simulink model "torqueBalancingYogaParametrizedForces2017"  (Simulink 9.0)
settings: Solver=FixedStepDiscrete  StartTime=0.0  StopTime="Config.SIMULATION_TIME "  FixedStep=Config.Ts  RelTol=1e-3  EnableMultiTasking=on
InitFcn:
  | cd(fileparts(which(bdroot)));
  | initTorqueBalancingYogaParametrized;
StopFcn:
  | cd(fileparts(which(bdroot)));
  | stopTorqueBalancingYoga;
undefined symbols (not defined in the file or in its folder): Config, delta_c, delta_x, delta_y, delta_z, DiscIntNeverNeededParam, Gain, Reg, ROBOT_DOF, ROBOT_DOF_FOR_SIMULINK, Sat, Sm
libraries: WBToolboxLibrary x85, simulink x4
(part 2 of 2)

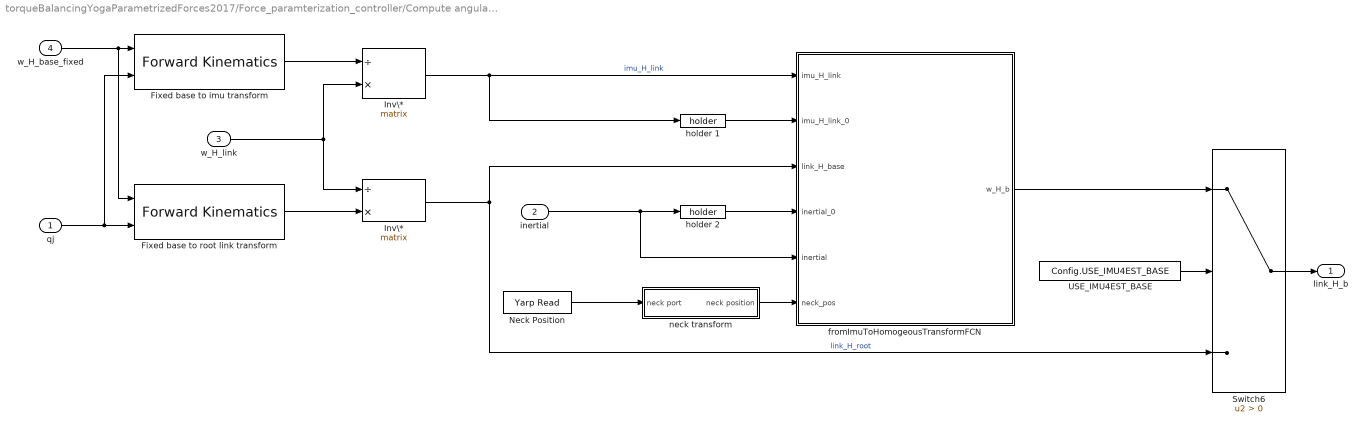
== system torqueBalancingYogaParametrizedForces2017/Force_paramterization_controller/Compute angular momentum integral/Compute base to fixed link transform/LFoot to base link transform  ==
  qj : Inport
  inertial : Inport  Port=2
  w_H_link : Inport  Port=3
  w_H_base_fixed : Inport  Port=4
  Fixed base to imu transform : WBToolboxLibrary/wholeBodyModel/Kinematics/Forward Kinematics  frameName=Frames.IMU
      settings: SourceProductName=Whole Body Toolbox
  Fixed base to root link transform : WBToolboxLibrary/wholeBodyModel/Kinematics/Forward Kinematics  frameName=Frames.BASE
      settings: SourceProductName=Whole Body Toolbox
  Inv\* : Product  Inputs=/*  Multiplication=Matrix(*)
  "Inv\\*  " : Product  Inputs=/*  Multiplication=Matrix(*)
  Neck Position : WBToolboxLibrary/Utilities/Yarp Read  portName=Ports.NECK_POS  signalSize=6  timeout=0.5  blocking=off  timestamp=off  autoconnect=on  errorOnConnection=off
      settings: SourceProductName=Whole Body Toolbox
  Switch6 : Switch  Criteria=u2 > Threshold
  USE_IMU4EST_BASE : Constant  Value=Config.USE_IMU4EST_BASE
  fromImuToHomogeousTransformFCN : MATLAB Function  TreatAsAtomicUnit=on
  holder 1 : WBToolboxLibrary/Utilities/holder 
      settings: SourceProductName=Whole Body Toolbox
  holder 2 : WBToolboxLibrary/Utilities/holder 
      settings: SourceProductName=Whole Body Toolbox
  neck transform : Subsystem
  link_H_b : Outport
  wires:
  Switch6/1 -> link_H_b/1
  "Inv\\*  "/1 -> Switch6/3, fromImuToHomogeousTransformFCN/3(link_H_base)  "link_H_root"
  USE_IMU4EST_BASE/1 -> Switch6/2
  Inv\*/1 -> fromImuToHomogeousTransformFCN/1(imu_H_link), holder 1/1  "imu_H_link"
  holder 2/1 -> fromImuToHomogeousTransformFCN/4(inertial_0)
  Fixed base to imu transform/1 -> Inv\*/1
  holder 1/1 -> fromImuToHomogeousTransformFCN/2(imu_H_link_0)
  qj/1 -> Fixed base to imu transform/2, Fixed base to root link transform/2
  fromImuToHomogeousTransformFCN/1(w_H_b) -> Switch6/1
  Fixed base to root link transform/1 -> "Inv\\*  "/2
  inertial/1 -> holder 2/1, fromImuToHomogeousTransformFCN/5(inertial)
  Neck Position/1 -> neck transform/1(neck port)
  neck transform/1(neck position) -> fromImuToHomogeousTransformFCN/6(neck_pos)
  w_H_link/1 -> "Inv\\*  "/1, Inv\*/2
  w_H_base_fixed/1 -> Fixed base to root link transform/1, Fixed base to imu transform/1

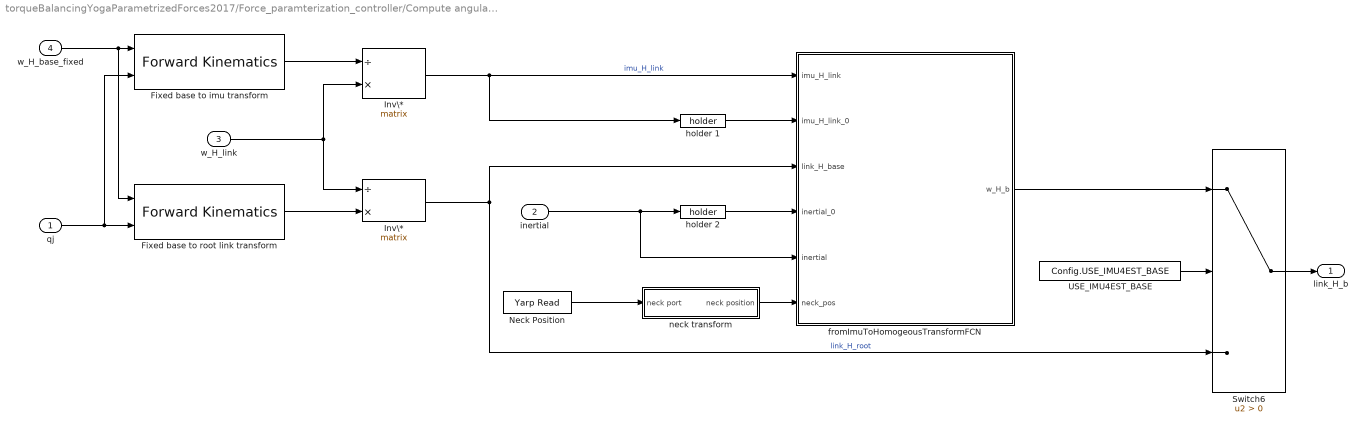
== system torqueBalancingYogaParametrizedForces2017/Force_paramterization_controller/Compute angular momentum integral/Compute base to fixed link transform/RFoot to base link transform ==
  qj : Inport
  inertial : Inport  Port=2
  w_H_link : Inport  Port=3
  w_H_base_fixed : Inport  Port=4
  Fixed base to imu transform : WBToolboxLibrary/wholeBodyModel/Kinematics/Forward Kinematics  frameName=Frames.IMU
      settings: SourceProductName=Whole Body Toolbox
  Fixed base to root link transform : WBToolboxLibrary/wholeBodyModel/Kinematics/Forward Kinematics  frameName=Frames.BASE
      settings: SourceProductName=Whole Body Toolbox
  Inv\* : Product  Inputs=/*  Multiplication=Matrix(*)
  "Inv\\*  " : Product  Inputs=/*  Multiplication=Matrix(*)
  Neck Position : WBToolboxLibrary/Utilities/Yarp Read  portName=Ports.NECK_POS  signalSize=6  timeout=0.5  blocking=off  timestamp=off  autoconnect=on  errorOnConnection=off
      settings: SourceProductName=Whole Body Toolbox
  Switch6 : Switch  Criteria=u2 > Threshold
  USE_IMU4EST_BASE : Constant  Value=Config.USE_IMU4EST_BASE
  fromImuToHomogeousTransformFCN : MATLAB Function  TreatAsAtomicUnit=on
  holder 1 : WBToolboxLibrary/Utilities/holder 
      settings: SourceProductName=Whole Body Toolbox
  holder 2 : WBToolboxLibrary/Utilities/holder 
      settings: SourceProductName=Whole Body Toolbox
  neck transform : Subsystem
  link_H_b : Outport
  wires:
  Switch6/1 -> link_H_b/1
  "Inv\\*  "/1 -> Switch6/3, fromImuToHomogeousTransformFCN/3(link_H_base)  "link_H_root"
  USE_IMU4EST_BASE/1 -> Switch6/2
  Inv\*/1 -> fromImuToHomogeousTransformFCN/1(imu_H_link), holder 1/1  "imu_H_link"
  holder 2/1 -> fromImuToHomogeousTransformFCN/4(inertial_0)
  Fixed base to imu transform/1 -> Inv\*/1
  holder 1/1 -> fromImuToHomogeousTransformFCN/2(imu_H_link_0)
  qj/1 -> Fixed base to imu transform/2, Fixed base to root link transform/2
  fromImuToHomogeousTransformFCN/1(w_H_b) -> Switch6/1
  Fixed base to root link transform/1 -> "Inv\\*  "/2
  inertial/1 -> holder 2/1, fromImuToHomogeousTransformFCN/5(inertial)
  Neck Position/1 -> neck transform/1(neck port)
  neck transform/1(neck position) -> fromImuToHomogeousTransformFCN/6(neck_pos)
  w_H_link/1 -> "Inv\\*  "/1, Inv\*/2
  w_H_base_fixed/1 -> Fixed base to root link transform/1, Fixed base to imu transform/1

== system torqueBalancingYogaParametrizedForces2017/Robot State and References/Internal Coordinator/Base to fixed_link/LFoot to base link transform  ==
  qj : Inport
  inertial : Inport  Port=2
  w_H_link : Inport  Port=3
  w_H_base_fixed : Inport  Port=4
  Fixed base to imu transform : WBToolboxLibrary/wholeBodyModel/Kinematics/Forward Kinematics  frameName=Frames.IMU
      settings: SourceProductName=Whole Body Toolbox
  Fixed base to root link transform : WBToolboxLibrary/wholeBodyModel/Kinematics/Forward Kinematics  frameName=Frames.BASE
      settings: SourceProductName=Whole Body Toolbox
  Inv\* : Product  Inputs=/*  Multiplication=Matrix(*)
  "Inv\\*  " : Product  Inputs=/*  Multiplication=Matrix(*)
  Neck Position : WBToolboxLibrary/Utilities/Yarp Read  portName=Ports.NECK_POS  signalSize=6  timeout=0.5  blocking=off  timestamp=off  autoconnect=on  errorOnConnection=off
      settings: SourceProductName=Whole Body Toolbox
  Switch6 : Switch  Criteria=u2 > Threshold
  USE_IMU4EST_BASE : Constant  Value=Config.USE_IMU4EST_BASE
  fromImuToHomogeousTransformFCN : MATLAB Function  TreatAsAtomicUnit=on
  holder 1 : WBToolboxLibrary/Utilities/holder 
      settings: SourceProductName=Whole Body Toolbox
  holder 2 : WBToolboxLibrary/Utilities/holder 
      settings: SourceProductName=Whole Body Toolbox
  neck transform : Subsystem
  link_H_b : Outport
  wires:
  Switch6/1 -> link_H_b/1
  "Inv\\*  "/1 -> Switch6/3, fromImuToHomogeousTransformFCN/3(link_H_base)  "link_H_root"
  USE_IMU4EST_BASE/1 -> Switch6/2
  Inv\*/1 -> fromImuToHomogeousTransformFCN/1(imu_H_link), holder 1/1  "imu_H_link"
  holder 2/1 -> fromImuToHomogeousTransformFCN/4(inertial_0)
  Fixed base to imu transform/1 -> Inv\*/1
  holder 1/1 -> fromImuToHomogeousTransformFCN/2(imu_H_link_0)
  qj/1 -> Fixed base to imu transform/2, Fixed base to root link transform/2
  fromImuToHomogeousTransformFCN/1(w_H_b) -> Switch6/1
  Fixed base to root link transform/1 -> "Inv\\*  "/2
  inertial/1 -> holder 2/1, fromImuToHomogeousTransformFCN/5(inertial)
  Neck Position/1 -> neck transform/1(neck port)
  neck transform/1(neck position) -> fromImuToHomogeousTransformFCN/6(neck_pos)
  w_H_link/1 -> "Inv\\*  "/1, Inv\*/2
  w_H_base_fixed/1 -> Fixed base to root link transform/1, Fixed base to imu transform/1

== system torqueBalancingYogaParametrizedForces2017/Robot State and References/Internal Coordinator/Compute State Velocity/Feet Jacobians ==
  qj : Inport
  w_H_b : Inport  Port=2
  Jacobian LFoot : WBToolboxLibrary/wholeBodyModel/Jacobians/Jacobian  frameName=Frames.LEFT_FOOT
      settings: SourceProductName=Whole Body Toolbox
  Jacobian RFoot : WBToolboxLibrary/wholeBodyModel/Jacobians/Jacobian  frameName=Frames.RIGHT_FOOT
      settings: SourceProductName=Whole Body Toolbox
  J_LFoot : Outport
  J_RFoot : Outport  Port=2
  wires:
  Jacobian LFoot/1 -> J_LFoot/1
  Jacobian RFoot/1 -> J_RFoot/1
  w_H_b/1 -> Jacobian RFoot/1, Jacobian LFoot/1
  qj/1 -> Jacobian LFoot/2, Jacobian RFoot/2

== system torqueBalancingYogaParametrizedForces2017/Robot State and References/State Machine Yoga/Compute State Velocity/Feet Jacobians ==
  qj : Inport
  w_H_b : Inport  Port=2
  Jacobian LFoot : WBToolboxLibrary/wholeBodyModel/Jacobians/Jacobian  frameName=Frames.LEFT_FOOT
      settings: SourceProductName=Whole Body Toolbox
  Jacobian RFoot : WBToolboxLibrary/wholeBodyModel/Jacobians/Jacobian  frameName=Frames.RIGHT_FOOT
      settings: SourceProductName=Whole Body Toolbox
  J_LFoot : Outport
  J_RFoot : Outport  Port=2
  wires:
  Jacobian LFoot/1 -> J_LFoot/1
  Jacobian RFoot/1 -> J_RFoot/1
  w_H_b/1 -> Jacobian RFoot/1, Jacobian LFoot/1
  qj/1 -> Jacobian LFoot/2, Jacobian RFoot/2

== system torqueBalancingYogaParametrizedForces2017/Robot State and References/State Machine Yoga/Compute base to fixed link transform/LFoot to base link transform  ==
  qj : Inport
  inertial : Inport  Port=2
  w_H_link : Inport  Port=3
  w_H_base_fixed : Inport  Port=4
  Fixed base to imu transform : WBToolboxLibrary/wholeBodyModel/Kinematics/Forward Kinematics  frameName=Frames.IMU
      settings: SourceProductName=Whole Body Toolbox
  Fixed base to root link transform : WBToolboxLibrary/wholeBodyModel/Kinematics/Forward Kinematics  frameName=Frames.BASE
      settings: SourceProductName=Whole Body Toolbox
  Inv\* : Product  Inputs=/*  Multiplication=Matrix(*)
  "Inv\\*  " : Product  Inputs=/*  Multiplication=Matrix(*)
  Neck Position : WBToolboxLibrary/Utilities/Yarp Read  portName=Ports.NECK_POS  signalSize=6  timeout=0.5  blocking=off  timestamp=off  autoconnect=on  errorOnConnection=off
      settings: SourceProductName=Whole Body Toolbox
  Switch6 : Switch  Criteria=u2 > Threshold
  USE_IMU4EST_BASE : Constant  Value=Config.USE_IMU4EST_BASE
  fromImuToHomogeousTransformFCN : MATLAB Function  TreatAsAtomicUnit=on
  holder 1 : WBToolboxLibrary/Utilities/holder 
      settings: SourceProductName=Whole Body Toolbox
  holder 2 : WBToolboxLibrary/Utilities/holder 
      settings: SourceProductName=Whole Body Toolbox
  neck transform : Subsystem
  link_H_b : Outport
  wires:
  Switch6/1 -> link_H_b/1
  "Inv\\*  "/1 -> Switch6/3, fromImuToHomogeousTransformFCN/3(link_H_base)  "link_H_root"
  USE_IMU4EST_BASE/1 -> Switch6/2
  Inv\*/1 -> fromImuToHomogeousTransformFCN/1(imu_H_link), holder 1/1  "imu_H_link"
  holder 2/1 -> fromImuToHomogeousTransformFCN/4(inertial_0)
  Fixed base to imu transform/1 -> Inv\*/1
  holder 1/1 -> fromImuToHomogeousTransformFCN/2(imu_H_link_0)
  qj/1 -> Fixed base to imu transform/2, Fixed base to root link transform/2
  fromImuToHomogeousTransformFCN/1(w_H_b) -> Switch6/1
  Fixed base to root link transform/1 -> "Inv\\*  "/2
  inertial/1 -> holder 2/1, fromImuToHomogeousTransformFCN/5(inertial)
  Neck Position/1 -> neck transform/1(neck port)
  neck transform/1(neck position) -> fromImuToHomogeousTransformFCN/6(neck_pos)
  w_H_link/1 -> "Inv\\*  "/1, Inv\*/2
  w_H_base_fixed/1 -> Fixed base to root link transform/1, Fixed base to imu transform/1

== system torqueBalancingYogaParametrizedForces2017/Robot State and References/State Machine Yoga/Compute base to fixed link transform/RFoot to base link transform ==
  qj : Inport
  inertial : Inport  Port=2
  w_H_link : Inport  Port=3
  w_H_base_fixed : Inport  Port=4
  Fixed base to imu transform : WBToolboxLibrary/wholeBodyModel/Kinematics/Forward Kinematics  frameName=Frames.IMU
      settings: SourceProductName=Whole Body Toolbox
  Fixed base to root link transform : WBToolboxLibrary/wholeBodyModel/Kinematics/Forward Kinematics  frameName=Frames.BASE
      settings: SourceProductName=Whole Body Toolbox
  Inv\* : Product  Inputs=/*  Multiplication=Matrix(*)
  "Inv\\*  " : Product  Inputs=/*  Multiplication=Matrix(*)
  Neck Position : WBToolboxLibrary/Utilities/Yarp Read  portName=Ports.NECK_POS  signalSize=6  timeout=0.5  blocking=off  timestamp=off  autoconnect=on  errorOnConnection=off
      settings: SourceProductName=Whole Body Toolbox
  Switch6 : Switch  Criteria=u2 > Threshold
  USE_IMU4EST_BASE : Constant  Value=Config.USE_IMU4EST_BASE
  fromImuToHomogeousTransformFCN : MATLAB Function  TreatAsAtomicUnit=on
  holder 1 : WBToolboxLibrary/Utilities/holder 
      settings: SourceProductName=Whole Body Toolbox
  holder 2 : WBToolboxLibrary/Utilities/holder 
      settings: SourceProductName=Whole Body Toolbox
  neck transform : Subsystem
  link_H_b : Outport
  wires:
  Switch6/1 -> link_H_b/1
  "Inv\\*  "/1 -> Switch6/3, fromImuToHomogeousTransformFCN/3(link_H_base)  "link_H_root"
  USE_IMU4EST_BASE/1 -> Switch6/2
  Inv\*/1 -> fromImuToHomogeousTransformFCN/1(imu_H_link), holder 1/1  "imu_H_link"
  holder 2/1 -> fromImuToHomogeousTransformFCN/4(inertial_0)
  Fixed base to imu transform/1 -> Inv\*/1
  holder 1/1 -> fromImuToHomogeousTransformFCN/2(imu_H_link_0)
  qj/1 -> Fixed base to imu transform/2, Fixed base to root link transform/2
  fromImuToHomogeousTransformFCN/1(w_H_b) -> Switch6/1
  Fixed base to root link transform/1 -> "Inv\\*  "/2
  inertial/1 -> holder 2/1, fromImuToHomogeousTransformFCN/5(inertial)
  Neck Position/1 -> neck transform/1(neck port)
  neck transform/1(neck position) -> fromImuToHomogeousTransformFCN/6(neck_pos)
  w_H_link/1 -> "Inv\\*  "/1, Inv\*/2
  w_H_base_fixed/1 -> Fixed base to root link transform/1, Fixed base to imu transform/1

== system torqueBalancingYogaParametrizedForces2017/Force_paramterization_controller/Compute angular momentum integral/Compute base to fixed link transform/LFoot to base link transform /neck transform ==
  neck port : Inport
  Constant : Constant  Value=zeros(3,1)
  Gain : Gain  Gain=pi/180
  Selector1 : Selector  InputPortWidth=6  IndexOptions=Index vector (dialog)  Indices=[1:3]  OutputSizes=1
  Switch : Switch  Criteria=u2 > Threshold
  USE_IMU4EST_BASE1 : Constant  Value=Config.CORRECT_NECK_IMU
  neck position : Outport
  wires:
  neck port/1 -> Gain/1
  USE_IMU4EST_BASE1/1 -> Switch/2
  Switch/1 -> neck position/1
  Gain/1 -> Selector1/1
  Constant/1 -> Switch/3
  Selector1/1 -> Switch/1  "neck pos"

== system torqueBalancingYogaParametrizedForces2017/Force_paramterization_controller/Compute angular momentum integral/Compute base to fixed link transform/RFoot to base link transform/neck transform ==
  neck port : Inport
  Constant : Constant  Value=zeros(3,1)
  Gain : Gain  Gain=pi/180
  Selector1 : Selector  InputPortWidth=6  IndexOptions=Index vector (dialog)  Indices=[1:3]  OutputSizes=1
  Switch : Switch  Criteria=u2 > Threshold
  USE_IMU4EST_BASE1 : Constant  Value=Config.CORRECT_NECK_IMU
  neck position : Outport
  wires:
  neck port/1 -> Gain/1
  USE_IMU4EST_BASE1/1 -> Switch/2
  Switch/1 -> neck position/1
  Gain/1 -> Selector1/1
  Constant/1 -> Switch/3
  Selector1/1 -> Switch/1  "neck pos"

== system torqueBalancingYogaParametrizedForces2017/Robot State and References/Internal Coordinator/Base to fixed_link/LFoot to base link transform /neck transform ==
  neck port : Inport
  Constant : Constant  Value=zeros(3,1)
  Gain : Gain  Gain=pi/180
  Selector1 : Selector  InputPortWidth=6  IndexOptions=Index vector (dialog)  Indices=[1:3]  OutputSizes=1
  Switch : Switch  Criteria=u2 > Threshold
  USE_IMU4EST_BASE1 : Constant  Value=Config.CORRECT_NECK_IMU
  neck position : Outport
  wires:
  neck port/1 -> Gain/1
  USE_IMU4EST_BASE1/1 -> Switch/2
  Switch/1 -> neck position/1
  Gain/1 -> Selector1/1
  Constant/1 -> Switch/3
  Selector1/1 -> Switch/1  "neck pos"

== system torqueBalancingYogaParametrizedForces2017/Robot State and References/State Machine Yoga/Compute base to fixed link transform/LFoot to base link transform /neck transform ==
  neck port : Inport
  Constant : Constant  Value=zeros(3,1)
  Gain : Gain  Gain=pi/180
  Selector1 : Selector  InputPortWidth=6  IndexOptions=Index vector (dialog)  Indices=[1:3]  OutputSizes=1
  Switch : Switch  Criteria=u2 > Threshold
  USE_IMU4EST_BASE1 : Constant  Value=Config.CORRECT_NECK_IMU
  neck position : Outport
  wires:
  neck port/1 -> Gain/1
  USE_IMU4EST_BASE1/1 -> Switch/2
  Switch/1 -> neck position/1
  Gain/1 -> Selector1/1
  Constant/1 -> Switch/3
  Selector1/1 -> Switch/1  "neck pos"

== system torqueBalancingYogaParametrizedForces2017/Robot State and References/State Machine Yoga/Compute base to fixed link transform/RFoot to base link transform/neck transform ==
  neck port : Inport
  Constant : Constant  Value=zeros(3,1)
  Gain : Gain  Gain=pi/180
  Selector1 : Selector  InputPortWidth=6  IndexOptions=Index vector (dialog)  Indices=[1:3]  OutputSizes=1
  Switch : Switch  Criteria=u2 > Threshold
  USE_IMU4EST_BASE1 : Constant  Value=Config.CORRECT_NECK_IMU
  neck position : Outport
  wires:
  neck port/1 -> Gain/1
  USE_IMU4EST_BASE1/1 -> Switch/2
  Switch/1 -> neck position/1
  Gain/1 -> Selector1/1
  Constant/1 -> Switch/3
  Selector1/1 -> Switch/1  "neck pos"

== matlab function Force_paramterization_controller/Compute angular momentum integral/Compute base to fixed link transform/LFoot to base link transform /fromImuToHomogeousTransformFCN ==
  data: imu_H_link input double; imu_H_link_0 input double; link_H_base input double; inertial_0 input double; inertial input double; neck_pos input double; w_H_b output double; Config parameter double
function w_H_b = worldToBaseTransformWithIMUFCN(imu_H_link,imu_H_link_0,link_H_base,inertial_0,inertial,neck_pos,Config)

    w_H_b = worldToBaseTransformWithIMU(imu_H_link,imu_H_link_0,link_H_base,inertial_0,inertial,neck_pos,Config);

end

== matlab function Robot State and References/Internal Coordinator/Base to fixed_link/LFoot to base link transform /fromImuToHomogeousTransformFCN ==
  data: imu_H_link input double; imu_H_link_0 input double; link_H_base input double; inertial_0 input double; inertial input double; neck_pos input double; w_H_b output double; Config parameter double
function w_H_b = worldToBaseTransformWithIMUFCN(imu_H_link,imu_H_link_0,link_H_base,inertial_0,inertial,neck_pos,Config)

    w_H_b = worldToBaseTransformWithIMU(imu_H_link,imu_H_link_0,link_H_base,inertial_0,inertial,neck_pos,Config);

end

== matlab function Robot State and References/State Machine Yoga/Compute base to fixed link transform/RFoot to base link transform/fromImuToHomogeousTransformFCN ==
  data: imu_H_link input double; imu_H_link_0 input double; link_H_base input double; inertial_0 input double; inertial input double; neck_pos input double; w_H_b output double; Config parameter double
function w_H_b = worldToBaseTransformWithIMUFCN(imu_H_link,imu_H_link_0,link_H_base,inertial_0,inertial,neck_pos,Config)

    w_H_b = worldToBaseTransformWithIMU(imu_H_link,imu_H_link_0,link_H_base,inertial_0,inertial,neck_pos,Config);

end

== matlab function Force_paramterization_controller/Compute angular momentum integral/Compute base to fixed link transform/RFoot to base link transform/fromImuToHomogeousTransformFCN ==
  data: imu_H_link input double; imu_H_link_0 input double; link_H_base input double; inertial_0 input double; inertial input double; neck_pos input double; w_H_b output double; Config parameter double
function w_H_b = worldToBaseTransformWithIMUFCN(imu_H_link,imu_H_link_0,link_H_base,inertial_0,inertial,neck_pos,Config)

    w_H_b = worldToBaseTransformWithIMU(imu_H_link,imu_H_link_0,link_H_base,inertial_0,inertial,neck_pos,Config);

end

== matlab function Robot State and References/Internal Coordinator/Compute State Velocity/Compute Base Velocity ==
  data: J_LeftFoot input double; J_RightFoot input double; feetInContact input double; nu_b output double; qjDot input double; Reg parameter double
function nu_b = computeBaseVelocityFCN(J_LeftFoot, J_RightFoot, feetInContact, qjDot, Reg)

    nu_b = computeBaseVelocity(J_LeftFoot, J_RightFoot, feetInContact, qjDot, Reg);
end

== matlab function Dynamics and Kinematics/Dynamics/Add motors reflected inertias/Add motor reflected inertias ==
  data: M input double; M_with_inertia output double; Config parameter double
function M_with_inertia = addMotorsInertiaFCN(M,Config)

    M_with_inertia = addMotorsInertia(M,Config);

end

== matlab function Robot State and References/State Machine Yoga/Compute State Velocity/Compute Base Velocity ==
  data: J_LeftFoot input double; J_RightFoot input double; feetInContact input double; nu_b output double; qjDot input double; Reg parameter double
function nu_b = computeBaseVelocityFCN(J_LeftFoot, J_RightFoot, feetInContact, qjDot, Reg)

    nu_b = computeBaseVelocity(J_LeftFoot, J_RightFoot, feetInContact, qjDot, Reg);
end

== matlab function Robot State and References/State Machine Yoga/Compute base to fixed link transform/LFoot to base link transform /fromImuToHomogeousTransformFCN ==
  data: imu_H_link input double; imu_H_link_0 input double; link_H_base input double; inertial_0 input double; inertial input double; neck_pos input double; w_H_b output double; Config parameter double
function w_H_b = worldToBaseTransformWithIMUFCN(imu_H_link,imu_H_link_0,link_H_base,inertial_0,inertial,neck_pos,Config)

    w_H_b = worldToBaseTransformWithIMU(imu_H_link,imu_H_link_0,link_H_base,inertial_0,inertial,neck_pos,Config);

end

== matlab function Force_paramterization_controller/Compute joint torques (motor reflected inertia)/(transpose(T*Gamma))^{-1}*I_m*(T*Gamma)^{-1} ==
  data: reflectedInertia output double; Config parameter double
function reflectedInertia  = computeMotorsInertiaFCN(Config)

    [reflectedInertia] = computeMotorsInertia(Config);

end

== matlab function Robot State and References/Internal Coordinator/Reference Generator CoM ==
  data: pos_CoM_0 input double; t input double; references_CoM output double; Config parameter double
function references_CoM = referenceGeneratorCoMFCN(pos_CoM_0, t, Config)

    references_CoM = referenceGeneratorCoM(pos_CoM_0, t, Config);
end

== matlab function Force_paramterization_controller/Parametrized Forces  ==
  data: delta_c input double; f output double; xi input double; delta_x input double; delta_y input double; delta_z input double; F output double
function [f,F] = fcn(delta_c, xi, delta_x, delta_y, delta_z)

 f_L = [(sqrt(delta_c))*(tanh(xi(1)))*(exp(xi(3)))/(1+(tanh(xi(2))^2))^0.5;
       (sqrt(delta_c))*(tanh(xi(2)))*(exp(xi(3)))/(1+(tanh(xi(1))^2))^0.5;
       exp(xi(3));
       delta_y*(tanh(xi(4)))*(exp(xi(3)));
       delta_x*(tanh(xi(5)))*(exp(xi(3)));
       delta_z*(tanh(xi(6)))*(exp(xi(3)))];

 F_L = [(sqrt(delta_c))*(exp(xi(3)))*(1-(tanh(xi(1)))^2)/(1+(tanh(xi(2)))^2)^0.5                             , (sqrt(delta_c))*(exp(xi(3)))*(tanh(xi(1)))*(tanh(xi(2)))*(-1+(tanh(xi(2)))^2)/(1+(tanh(xi(2)))^2)^1.5, (sqrt(delta_c))*(exp(xi(3)))*(tanh(xi(1)))/(1+(tanh(xi(2)))^2)^0.5, 0                                       , 0                                       , 0;
        (sqrt(delta_c))*(exp(xi(3)))*(tanh(xi(1)))*(tanh(xi(2)))*(-1+(tanh(xi(1)))^2)/(1+(tanh(xi(1)))^2)^1.5, (sqrt(delta_c))*(exp(xi(3)))*(1-(tanh(xi(2)))^2)/(1+(tanh(xi(1)))^2)^0.5                             , (sqrt(delta_c))*(exp(xi(3)))*(tanh(xi(2)))/(1+(tanh(xi(1)))^2)^0.5, 0                                       , 0                                       , 0;
        0                                                                                                    , 0                                                                                                    , exp(xi(3))                                                        , 0                                       , 0                                       , 0;
        0                                                                                                    , 0                                                                                                    , delta_y*(tanh(xi(4)))*(exp(xi(3)))                                , delta_y*(1-(tanh(xi(4)))^2)*(exp(xi(3))), 0                                       , 0;
        0                                                                                                    , 0                                                                                                    , delta_x*(tanh(xi(5)))*(exp(xi(3)))                                , 0                                       , delta_x*(1-(tanh(xi(5)))^2)*(exp(xi(3))), 0;
        0                                                                                                    , 0                                                                                                    , delta_z*(tanh(xi(6)))*(exp(xi(3)))                                , 0                                       , 0                                       , delta_z*(1-(tanh(xi(6)))^2)*(exp(xi(3)))];                 
     
 f_R = [(sqrt(delta_c))*(tanh(xi(7)))*(exp(xi(9)))/(1+(tanh(xi(8))^2))^0.5;
       (sqrt(delta_c))*(tanh(xi(8)))*(exp(xi(9)))/(1+(tanh(xi(7))^2))^0.5;
       exp(xi(9));
       delta_y*(tanh(xi(10)))*(exp(xi(9)));
       delta_x*(tanh(xi(11)))*(exp(xi(9)));
       delta_z*(tanh(xi(12)))*(exp(xi(9)))];

 F_R = [(sqrt(delta_c))*(exp(xi(9)))*(1-(tanh(xi(7)))^2)/(1+(tanh(xi(8)))^2)^0.5                             , (sqrt(delta_c))*(exp(xi(9)))*(tanh(xi(7)))*(tanh(xi(8)))*(-1+(tanh(xi(8)))^2)/(1+(tanh(xi(8)))^2)^1.5, (sqrt(delta_c))*(exp(xi(9)))*(tanh(xi(7)))/(1+(tanh(xi(8)))^2)^0.5, 0                                        , 0                                        , 0;
        (sqrt(delta_c))*(exp(xi(9)))*(tanh(xi(7)))*(tanh(xi(8)))*(-1+(tanh(xi(7)))^2)/(1+(tanh(xi(7)))^2)^1.5, (sqrt(delta_c))*(exp(xi(9)))*(1-(tanh(xi(8)))^2)/(1+(tanh(xi(7)))^2)^0.5                             , (sqrt(delta_c))*(exp(xi(9)))*(tanh(xi(8)))/(1+(tanh(xi(7)))^2)^0.5, 0                                        , 0                                        , 0;
        0                                                                                                    , 0                                                                                                    , exp(xi(9))                                                        , 0                                        , 0                                        , 0;
        0                                                                                                    , 0                                                                                                    , delta_y*(tanh(xi(10)))*(exp(xi(9)))                               , delta_y*(1-(tanh(xi(10)))^2)*(exp(xi(9))), 0                                        , 0;
        0                                                                                                    , 0                                                                                                    , delta_x*(tanh(xi(11)))*(exp(xi(9)))                               , 0                                        , delta_x*(1-(tanh(xi(11)))^2)*(exp(xi(9))), 0;
        0                                                                                                    , 0                                                                                                    , delta_z*(tanh(xi(12)))*(exp(xi(9)))                               , 0                                        , 0                                        , delta_z*(1-(tanh(xi(12)))^2)*(exp(xi(9)))];                 
     
 
 f = [f_L ; f_R];
 F = [F_L, F_R];

== matlab function Robot State and References/State Machine Yoga/stateMachineYogaParametrizedFCN ==
  data: wrench_rightFoot input double; wrench_leftFoot input double; w_H_b output double; CoM_des output double; qj_des output double; constraints output double; CoM_0 input double; q0 input double; l_sole_CoM input double; r_sole_CoM input double; qj input double; t input double; l_sole_H_b input double; r_sole_H_b input double; Sm parameter double; impedances output double; KPCoM output double; KDCoM output double; KICoM output double; Gain parameter double; currentState output double; jointsSmoothingTime output double
function [w_H_b, CoM_des, qj_des, constraints, impedances, KPCoM, KDCoM, KICoM, currentState, jointsSmoothingTime] = ...
          stateMachineYogaParametrizedFCN(wrench_rightFoot, wrench_leftFoot, CoM_0, q0, l_sole_CoM, r_sole_CoM, qj, t, l_sole_H_b, r_sole_H_b, Sm, Gain)
 
         [w_H_b, CoM_des, qj_des, constraints, impedances, KPCoM, KDCoM, KICoM, currentState, jointsSmoothingTime] = ...
          stateMachineYogaParametrized(wrench_rightFoot, wrench_leftFoot, CoM_0, q0, l_sole_CoM, r_sole_CoM, qj, t, l_sole_H_b, r_sole_H_b, Sm, Gain); 
end

== matlab function Force_paramterization_controller/Momentum jerk Controller  ==
  data: SM_TYPE input double; tau_star output double; constraints input double; ROBOT_DOF_FOR_SIMULINK input double; qj input double; qjDes input double; nu input double; M input double; h input double; L input double; intHw input double; w_H_l_sole input double; w_H_r_sole input double; JL input double; JR input double; dJLv input double; dJRv input double; xCoM input double; J_CoM input double; desired_x_dx_ddx_CoM input double; gainsPCOM input double; gainsDCOM input double; gainsICOM input double; impedances input double; errorCoM output double; f_desired output double; Gain parameter double; Reg parameter double; xi_dot output double; Left_Right_F_T_Sensors input double; f input double; F input double; xi input double; state input double
function [tau_star, errorCoM, f_desired, xi_dot] = ...
              balancingControllerYogaParametrziedFCN(SM_TYPE, constraints, ROBOT_DOF_FOR_SIMULINK, qj, qjDes, nu, M, h, L, intHw, w_H_l_sole, w_H_r_sole, JL, JR, dJLv, dJRv, xCoM, J_CoM, desired_x_dx_ddx_CoM, ...
                  gainsPCOM, gainsDCOM, gainsICOM, impedances, Gain, Reg, Left_Right_F_T_Sensors, f, F, xi, state)
          
         [tau_star, errorCoM, f_desired, xi_dot] = ...
              balancingControllerYogaParametrized(SM_TYPE, constraints, ROBOT_DOF_FOR_SIMULINK, qj, qjDes, nu, M, h, L, intHw, w_H_l_sole, w_H_r_sole, JL, JR, dJLv, dJRv, xCoM, J_CoM, desired_x_dx_ddx_CoM, ...
                  gainsPCOM, gainsDCOM, gainsICOM, impedances, Gain, Reg, Left_Right_F_T_Sensors, f, F, xi, state);
end

== matlab function emergency stop: joint limits/MATLAB Function ==
  data: umin input double; umax input double; u input double; inRange output double; tol input double
function inRange = checkRangeFCN(umin, umax, u, tol)

     inRange = checkRange(umin, umax, u, tol);
end

== matlab function Force_paramterization_controller/Compute angular momentum integral/choose base to world transform ==
  data: state input double; booleanState output double
function booleanState = footOnGround(state)

    % output: a boolean variable whose value is 1 if the foot on ground is left
    % foot, and 0 if the foot on ground is the right foot. If both feet are on
    % ground, the variable is setted to 1.

    % states in which right foot is on ground: 9,10,11,12
    booleanState = 1;

    if state == 9 || state == 10 || state == 11 || state == 12

        booleanState = 0;
    end
end

== matlab function Force_paramterization_controller/Compute angular momentum integral/References for H ==
  data: qjErr input double; JL input double; JR input double; nu_b_equivalent output double; Reg parameter double; activeFeetConstraints input double
function nu_b_equivalent = generateReferencesForH_FCN(qjErr, JL, JR, Reg, activeFeetConstraints)

    if activeFeetConstraints(1) == 1
    
        pinvJb          = (JL(:,1:6)'*JL(:,1:6) + Reg.pinvDamp_nu_b*eye(6))\JL(:,1:6)';
        nu_b_equivalent = -pinvJb*JL(:,7:end)*qjErr;
    else
    
        pinvJb          = (JR(:,1:6)'*JR(:,1:6) + Reg.pinvDamp_nu_b*eye(6))\JR(:,1:6)';
        nu_b_equivalent = -pinvJb*JR(:,7:end)*qjErr;
    end
end
